simulink model "GS_model"  (R2018b)
settings: Solver=ode5  StartTime=0.0  StopTime=SimuStopTime  FixedStep=T_Simu  RelTol=1e-3
InitFcn:
  | Initial
undefined symbols (not defined in the file or in its folder): Aba10, Aba20, aeroCIP2006_S, aeroCIP2006_X, aeroCIP2006_Y, Agl0, Ass_kS, Ass_n1, Ass_n2, Ass_n3, Ass_n4, Ass_Noise, Ass_R, Ass_Resolution, Ass_TmOrder, AssA_Fix_Abs, AssB_Fix_Abs, AssC_Fix_Abs, AssD_Fix_Abs, AssE_Fix_Aps, AssF_Fix_Aps, C, c_max, c_min, Cd, CenterOfFigNX, CenterOfFigNY, CenterOfFigNZ, CenterOfFigP1, CenterOfFigP2, CenterOfFigPX, CenterOfFigPY, CenterOfFigPZ, Cmu, Crou, DEG2RAD, DiscIntNeverNeededParam, Eg_Dir, Eg_F, Eg_PrepareTime, Eg_r_L_L, Fw_Abf, Fw_Hmax, Fw_J, Fw_Spd0, Fw_Tmax, git_hash_BaseLine, git_hash_Project, Gnss_Noise_Pos, Gnss_Noise_Vel, Gnss_PropgationTime, GyroA_Fix_Abg, GyroA_Noise, GyroB_Fix_Abg, GyroB_Noise, GyroC_Fix_Abg, GyroC_Noise, GyroD_Fix_Abg, GyroD_Noise, h ... (+94)
libraries: simulink x308, sharedutil x46, aerolibutil x37, sharedtransform x31, vrlib x14, aerolibgravity2 x2
(part 7 of 20)

== system GS_model/Subsystem2/Subsystem/PhysicsModel/Environment/Air Torque Subsystem/Subsystem ==
  Sun Vector in J2000 : Inport
  Earth Vector in J2000 : Inport  Port=2
  Add : Sum
  Demux : Demux  Outputs=3
  Dot Product : DotProduct  InputSameDT=on  OutDataTypeStr=Inherit: Inherit via internal rule
  Dot Product1 : DotProduct  InputSameDT=on  OutDataTypeStr=Inherit: Inherit via internal rule
  Fcn : Fcn  Expr=sqrt(u(1)^2+u(2)^2)
  Gain : Gain  Gain=1e-9
  MATLAB Function : MATLAB Function  TreatAsAtomicUnit=on
  MATLAB Function1 : MATLAB Function  TreatAsAtomicUnit=on
  Math Function : Math  Operator=pow  SaturateOnIntegerOverflow=on
  Mux : Mux  Inputs=3
  Product : Product  Inputs=**/
  Product1 : Product  Inputs=**
  Product2 : Product  Inputs=**
  Product3 : Product  Inputs=**
  Saturation : Saturate  UpperLimit=2000000  LowerLimit=200000
  Sqrt : Sqrt  SaturateOnIntegerOverflow=on
  Terminator : Terminator
  Terminator1 : Terminator
  Trigonometric Function : Trigonometry  Operator=cos
  Trigonometric Function1 : Trigonometry
  Trigonometric Function2 : Trigonometry  Operator=cos
  Trigonometric Function3 : Trigonometry
  c_psi1 : Sum  Inputs=-+
  c_psi2 : Sum
  c_psi3 : Sum
  declination of sun : Trigonometry  Operator=atan2
  h : Constant  Value=h
  h1 : Constant  Value=c_min
  h2 : Constant  Value=c_max
  right ascension of sun : Trigonometry  Operator=atan2
  sun_delay : Constant  Value=ra_lag
  sun_delay2 : Constant  Value=0.5
  sun_delay3 : Constant  Value=n_prm
  rou : Outport
  wires:
  Demux/3 -> declination of sun/1
  Fcn/1 -> declination of sun/2
  Sun Vector in J2000/1 -> Fcn/1, Demux/1
  Demux/1 -> right ascension of sun/2
  Demux/2 -> right ascension of sun/1
  h2/1 -> MATLAB Function1/4(c_max)
  MATLAB Function/2(lat) -> Terminator1/1
  Product3/1 -> c_psi3/2
  Math Function/1 -> Product3/1
  c_psi3/1 -> Gain/1
  Gain/1 -> rou/1
  Product1/1 -> Mux/1
  c_psi2/1 -> Math Function/1
  Trigonometric Function1/1 -> Product2/1
  Sqrt/1 -> Product/3
  sun_delay2/1 -> c_psi2/1, Product/1
  Dot Product1/1 -> Sqrt/1
  Dot Product/1 -> Product/2
  MATLAB Function/3(h) -> Saturation/1
  Mux/1 -> Dot Product/1
  Saturation/1 -> MATLAB Function1/1(height)
  Trigonometric Function/1 -> Product1/1
  Trigonometric Function3/1 -> Mux/3
  Product2/1 -> Mux/2
  Trigonometric Function2/1 -> Product2/2, Product1/2
  MATLAB Function1/2(d_max) -> c_psi1/2
  MATLAB Function1/1(d_min) -> c_psi3/1, c_psi1/1
  c_psi1/1 -> Product3/2
  declination of sun/1 -> Trigonometric Function3/1, Trigonometric Function2/1
  Add/1 -> Trigonometric Function1/1, Trigonometric Function/1
  Product/1 -> c_psi2/2
  h/1 -> MATLAB Function1/2(h)
  h1/1 -> MATLAB Function1/3(c_min)
  sun_delay/1 -> Add/1
  right ascension of sun/1 -> Add/2
  sun_delay3/1 -> Math Function/2
  Earth Vector in J2000/1 -> Dot Product1/1, Dot Product/2, Dot Product1/2, MATLAB Function/1(r)
  MATLAB Function/1(lon) -> Terminator/1

== system GS_model/Subsystem2/Subsystem/PhysicsModel/Environment/Air Torque Subsystem/satalite board ==
  "[Vs]b" : Inport
  Fa' : Inport  Port=2
  Abp_PY : Inport  Port=3
  Abp_NY : Inport  Port=4
  Cent : Inport  Port=5
  UnlockSpread : Inport  Port=6
  +Y SolarPanel : Subsystem
  -Y SolarPanel : Subsystem
  Demux : Demux  Outputs=2
  Product{1..4} (4 alike) : Product  SaturateOnIntegerOverflow=on  OutDataTypeStr=Inherit: Same as first input
  Sum1 : Sum  Inputs=+++++
  Sum2 : Sum  Inputs=+++++
  "Torque from  board perpendicular to z axis " : Subsystem  TreatAsAtomicUnit=on
  Torque from board perpendicular to x axis : Subsystem  TreatAsAtomicUnit=on
  Torque from board perpendicular to y axis : Subsystem  TreatAsAtomicUnit=on
  F_a(b) : Outport
  T_a(b) : Outport  Port=2
  wires:
  "[Vs]b"/1 -> Torque from board perpendicular to x axis/1(vs(b)), Torque from board perpendicular to y axis/1(vs(b)), "Torque from  board perpendicular to z axis "/1("[Vs]b_nor"), +Y SolarPanel/1(vs(b)), -Y SolarPanel/1(vs(b))
  Fa'/1 -> Torque from board perpendicular to x axis/2(Fa'), Torque from board perpendicular to y axis/2(Fa'), "Torque from  board perpendicular to z axis "/2(Fa'), +Y SolarPanel/2(Fa'), -Y SolarPanel/2(Fa')
  Abp_PY/1 -> +Y SolarPanel/3("Abp ")
  Torque from board perpendicular to x axis/1(Tx) -> Sum1/1
  Sum1/1 -> T_a(b)/1
  Torque from board perpendicular to y axis/1(Ty) -> Sum1/2
  "Torque from  board perpendicular to z axis "/1(Tz) -> Sum1/3
  "Torque from  board perpendicular to z axis "/2(Fz) -> Sum2/3
  Torque from board perpendicular to y axis/2(Fy) -> Sum2/2
  Torque from board perpendicular to x axis/2(Fx) -> Sum2/1
  Sum2/1 -> F_a(b)/1
  Abp_NY/1 -> -Y SolarPanel/3("Abp ")
  Cent/1 -> Torque from board perpendicular to x axis/3(Cent), Torque from board perpendicular to y axis/3(Cent), +Y SolarPanel/4(Cent), -Y SolarPanel/4(Cent), "Torque from  board perpendicular to z axis "/3(Cent)
  Product2/1 -> Sum1/5
  Product4/1 -> Sum2/5
  +Y SolarPanel/2("F_panel ") -> Product3/1
  Product3/1 -> Sum2/4
  +Y SolarPanel/1("T_panel ") -> Product1/1
  Product1/1 -> Sum1/4
  -Y SolarPanel/1("T_panel ") -> Product2/2
  -Y SolarPanel/2("F_panel ") -> Product4/2
  UnlockSpread/1 -> Demux/1
  Demux/1 -> Product1/2, Product3/2
  Demux/2 -> Product4/1, Product2/1

== system GS_model/Subsystem2/Subsystem/PhysicsModel/Environment/MagneticCal/Subsystem1 ==
  LB_Geocentric : Inport
  Orbit : Inport  Port=2
  Aop1 : Subsystem
  Constant : Constant  Value=pi/2
  Divide : Product  Inputs=*/
  Fcn : Fcn  Expr=u(3)
  Fcn1 : Fcn  Expr=u(2)
  Fcn2 : Fcn  Expr=u(5)+u(6)
  Gain : Gain  Gain=-1
  If : If
  If Action Subsystem : Subsystem  TreatAsAtomicUnit=on
  If Action Subsystem1 : Subsystem  TreatAsAtomicUnit=on
  Merge : Merge
  Saturation : Saturate  UpperLimit=1  LowerLimit=-1
  Sum : Sum  Inputs=|-+
  Trigonometric Function : Trigonometry
  Trigonometric Function1 : Trigonometry  Operator=cos
  Trigonometric Function2 : Trigonometry  Operator=asin
  Trigonometric Function3 : Trigonometry  Operator=cos
  Aop : Outport
  wires:
  Trigonometric Function1/1 -> Gain/1
  Fcn/1 -> Trigonometric Function1/1  "i"
  Orbit/1 -> Fcn2/1, Fcn/1
  Constant/1 -> Sum/2
  Sum/1 -> Trigonometric Function/1
  Merge/1 -> Aop1/1(In1)
  Trigonometric Function/1 -> Divide/2
  If Action Subsystem1/1(Out1) -> Merge/2
  If/2 -> If Action Subsystem1/Action
  Fcn1/1 -> Sum/1
  If Action Subsystem/1(Out1) -> Merge/1
  Trigonometric Function3/1 -> If/1
  If/1 -> If Action Subsystem/Action
  Trigonometric Function2/1 -> If Action Subsystem1/1(In1), If Action Subsystem/1(In1)
  Fcn2/1 -> Trigonometric Function3/1  "u"
  Divide/1 -> Saturation/1
  Aop1/1(Out1) -> Aop/1
  Gain/1 -> Divide/1
  LB_Geocentric/1 -> Fcn1/1
  Saturation/1 -> Trigonometric Function2/1

== system GS_model/Subsystem2/Subsystem/PhysicsModel/Environment/Sun  press torque/Panel Angle ==
  Sun(b) : Inport
  Constant1 : Constant  Value=0
  Constant4 : Constant  Value=[0;0;-1]
  Demux : Demux  Outputs=3
  Divide1 : Product  Inputs=*/
  Dot Product : DotProduct  InputSameDT=on  OutDataTypeStr=Inherit: Inherit via internal rule
  Fcn2 : Fcn  Expr=sqrt(u(1)^2+u(2)^2+u(3)^2)
  Fcn3 : Fcn  Expr=u(1)
  If : If
  If Action Subsystem : Subsystem  TreatAsAtomicUnit=on
  If Action Subsystem1 : Subsystem  TreatAsAtomicUnit=on
  Merge : Merge
  Mux : Mux  Inputs=3
  Terminator : Terminator
  Trigonometric Function1 : Trigonometry  Operator=acos
  PanelAngle : Outport
  wires:
  Mux/1 -> Fcn2/1, Divide1/1
  Demux/3 -> Mux/3
  Constant1/1 -> Mux/2
  Demux/2 -> Terminator/1
  Demux/1 -> Mux/1
  Constant4/1 -> Dot Product/2
  Merge/1 -> PanelAngle/1
  Divide1/1 -> Fcn3/1, Dot Product/1
  Fcn3/1 -> If/1
  If/1 -> If Action Subsystem/Action
  If/2 -> If Action Subsystem1/Action
  If Action Subsystem/1(Out1) -> Merge/1
  If Action Subsystem1/1(Out1) -> Merge/2
  Fcn2/1 -> Divide1/2
  Trigonometric Function1/1 -> If Action Subsystem1/1(In1), If Action Subsystem/1(In1)
  Dot Product/1 -> Trigonometric Function1/1
  Sun(b)/1 -> Demux/1

== system GS_model/Subsystem2/Subsystem/PhysicsModel/Environment/Sun  press torque/Sun  press torque2 ==
  UnlockSpread : Inport
  Abp_PY : Inport  Port=2
  Abp_NY : Inport  Port=3
  Cent : Inport  Port=4
  IfSeeSun : Inport  Port=5
  TC_SunPressCoeff : Inport  Port=6
  Sun(b) : Inport  Port=7
  If Action Subsystem3 : Subsystem  TreatAsAtomicUnit=on
  If1 : If  IfExpression=u1 ==1
  Merge1 : Merge
  Merge3 : Merge
  Sun  press torque : Subsystem  TreatAsAtomicUnit=on
  F_sun : Outport
  T_sun : Outport  Port=2
  wires:
  If1/1 -> Sun  press torque/Action
  If1/2 -> If Action Subsystem3/Action
  Sun(b)/1 -> Sun  press torque/1(sun(b))
  Abp_PY/1 -> Sun  press torque/2(Abp_PY)
  If Action Subsystem3/2(T_sun) -> Merge3/2
  Sun  press torque/1(T_sun) -> Merge3/1
  Sun  press torque/2(F_sun) -> Merge1/1
  If Action Subsystem3/1(F_sun) -> Merge1/2
  Merge1/1 -> F_sun/1
  Merge3/1 -> T_sun/1
  IfSeeSun/1 -> If1/1
  Abp_NY/1 -> Sun  press torque/3(Abp_NY)
  Cent/1 -> Sun  press torque/4(Cent)
  UnlockSpread/1 -> Sun  press torque/5(UnlockSpread)
  TC_SunPressCoeff/1 -> Sun  press torque/6(TC_SunPressCoeff)

== system GS_model/Subsystem2/Subsystem/PhysicsModel/Environment/SunshineAreaCal/If Action Subsystem2 ==
  Action Port : ActionPort  ActionType=then
  Constant : Constant  Value=0
  Shadow : Outport  InitialOutput=0
  wires:
  Constant/1 -> Shadow/1

== system GS_model/Subsystem2/Subsystem/PhysicsModel/Environment/SunshineAreaCal/If Action Subsystem5 ==
  Action Port : ActionPort  ActionType=else
  Constant : Constant
  Sunshine : Outport  InitialOutput=1
  wires:
  Constant/1 -> Sunshine/1

== system GS_model/Subsystem2/Subsystem/PhysicsModel/Orbit/Compute osculating elements/  ==
  note: 0<=OMG<=2pi
  Hi : Inport
  Constant : Constant  Value=0
  Constant1 : Constant  Value=[1;0;0]
  Fcn1 : Fcn  Expr=u(1)
  Fcn2 : Fcn  Expr=u(2)
  If : If  IfExpression=u1 < 0
  If Action Subsystem : Subsystem  TreatAsAtomicUnit=on
  If Action Subsystem1 : Subsystem  TreatAsAtomicUnit=on
  MatrixMultiply : Product  Multiplication=Matrix(*)
  Merge : Merge
  Mux : Mux  Inputs=3
  Mux3 : Mux  Inputs=2
  Rotation Angles to Direction Cosine Matrix : sharedtransform/Rotation Angles to Direction Cosine Matrix  rotationOrder=ZYX  aMode=aMode
      settings: SourceProductBaseCode=AE,PW,MT,VE,VP
  Transpose : Math  Operator=transpose  SaturateOnIntegerOverflow=on
  tg(OMG)=Hxi/(-Hyi) : Fcn  Expr=atan2(u[1],-u[2])
  OMG : Outport
  N : Outport  Port=2
  wires:
  Fcn1/1 -> Mux3/1
  Fcn2/1 -> Mux3/2
  Mux3/1 -> tg(OMG)=Hxi/(-Hyi)/1
  tg(OMG)=Hxi/(-Hyi)/1 -> If/1, If Action Subsystem/1(In1), Mux/1, If Action Subsystem1/1(In1)
  If/1 -> If Action Subsystem/Action
  If/2 -> If Action Subsystem1/Action
  If Action Subsystem/1(Out1) -> Merge/1
  If Action Subsystem1/1(Out1) -> Merge/2
  Merge/1 -> OMG/1
  Hi/1 -> Fcn1/1, Fcn2/1
  Constant/1 -> Mux/2, Mux/3
  Mux/1 -> Rotation Angles to Direction Cosine Matrix/1
  Rotation Angles to Direction Cosine Matrix/1 -> Transpose/1
  Constant1/1 -> MatrixMultiply/2
  MatrixMultiply/1 -> N/1
  Transpose/1 -> MatrixMultiply/1

== system GS_model/Subsystem2/Subsystem/PhysicsModel/Orbit/Compute osculating elements/      ==
  N : Inport
  R_xyz : Inport  Port=2
  Divide : Product  Inputs=*/
  Dot Product4 : DotProduct  InputSameDT=on  OutDataTypeStr=Inherit: Inherit via internal rule
  Fcn3 : Fcn  Expr=sqrt(u[1]^2+u[2]^2+u[3]^2)
  Fcn4 : Fcn  Expr=u[3]
  If Action Subsystem2 : Subsystem  TreatAsAtomicUnit=on
  If Action Subsystem3 : Subsystem  TreatAsAtomicUnit=on
  If1 : If
  Merge1 : Merge
  Trigonometric Function : Trigonometry  Operator=acos
  u : Outport
  wires:
  N/1 -> Dot Product4/1
  R_xyz/1 -> Fcn3/1, Dot Product4/2, Fcn4/1
  Divide/1 -> Trigonometric Function/1
  Fcn4/1 -> If1/1
  If1/1 -> If Action Subsystem2/Action
  Trigonometric Function/1 -> If Action Subsystem2/1(In1), If Action Subsystem3/1(In1)
  If Action Subsystem2/1(Out1) -> Merge1/1
  If Action Subsystem3/1(Out1) -> Merge1/2
  Merge1/1 -> u/1
  If1/2 -> If Action Subsystem3/Action
  Dot Product4/1 -> Divide/1
  Fcn3/1 -> Divide/2

== system GS_model/Subsystem2/Subsystem/PhysicsModel/Orbit/Compute osculating elements/   1 ==
  note: e
  note: 0<=omg<=2pi
  H_xyz : Inport
  V_xyz : Inport  Port=2
  R_xyz : Inport  Port=3
  OMG : Inport  Port=4
  i : Inport  Port=5
  3x3 Cross Product1 : sharedutil/3x3 Cross Product  aMode=aMode
      settings: SourceProductBaseCode=AE,PW,MT,VE,VP
  Constant1 : Constant  Value=0
  Demux : Demux  Outputs=3
  Divide : Product  Inputs=*/
  Fcn3 : Fcn  Expr=sqrt(u[1]^2+u[2]^2+u[3]^2)
  Gain3 : Gain  Gain=1/miu  SaturateOnIntegerOverflow=on  OutDataTypeStr=Inherit: Same as input  ParamDataTypeStr=Inherit: Same as input
  If : If  IfExpression=u1 >= 0
  If Action Subsystem : Subsystem  TreatAsAtomicUnit=on
  If Action Subsystem1 : Subsystem  TreatAsAtomicUnit=on
  MatrixMultiply : Product  Multiplication=Matrix(*)
  Merge : Merge
  Mux1 : Mux  Inputs=3
  Rotation Angles to Direction Cosine Matrix : sharedtransform/Rotation Angles to Direction Cosine Matrix  rotationOrder=ZXY  aMode=aMode
      settings: SourceProductBaseCode=AE,PW,MT,VE,VP
  Sum : Sum  Inputs=|--  SaturateOnIntegerOverflow=on
  Terminator : Terminator
  Trigonometric Function : Trigonometry  Operator=atan2
  omg : Outport
  wires:
  H_xyz/1 -> 3x3 Cross Product1/1
  If Action Subsystem1/1(Out1) -> Merge/2
  If Action Subsystem/1(Out1) -> Merge/1
  Trigonometric Function/1 -> If/1, If Action Subsystem1/1(In1), If Action Subsystem/1(In1)
  Sum/1 -> MatrixMultiply/2
  Divide/1 -> Sum/2
  Fcn3/1 -> Divide/2
  3x3 Cross Product1/1 -> Gain3/1
  V_xyz/1 -> 3x3 Cross Product1/2
  Merge/1 -> omg/1
  If/1 -> If Action Subsystem/Action
  If/2 -> If Action Subsystem1/Action
  R_xyz/1 -> Divide/1, Fcn3/1
  Gain3/1 -> Sum/1
  Rotation Angles to Direction Cosine Matrix/1 -> MatrixMultiply/1
  Mux1/1 -> Rotation Angles to Direction Cosine Matrix/1
  OMG/1 -> Mux1/1
  i/1 -> Mux1/2
  Constant1/1 -> Mux1/3
  MatrixMultiply/1 -> Demux/1
  Demux/2 -> Trigonometric Function/1
  Demux/1 -> Trigonometric Function/2
  Demux/3 -> Terminator/1

== system GS_model/Subsystem2/Subsystem/Sensor/Ass/BodyAss(A&B&C&D)Model/Subsystem ==
  note: TC_AssGNDSet[6*1]
  note: TC_AssErr_Constant[2*1]
  note: TC_AssErr_WildValue[2*1]
  note: TC_AssErr_Jump[4*1]
  note: TC_AssErr_Wave[3*1]
  Sunshine : Inport
  AbAss : Inport  Port=2
  Sun_b : Inport  Port=3
  kS_Ass : Inport  Port=4
  TC_Ass : Inport  Port=5
  AssNum : Inport  Port=6
  AssErrModel : Subsystem
      mask Display: disp('AssErrModel')
  AssMathModel : Subsystem
      mask Display: disp('AssMathModel')
  Demux : Demux  Outputs=[6;2;2;4;3]
  TM_Data_AssA : Outport
  wires:
  Sunshine/1 -> AssMathModel/1(Sunshine)
  AbAss/1 -> AssMathModel/2(AbAss)
  Sun_b/1 -> AssMathModel/3(Sun_b)
  kS_Ass/1 -> AssMathModel/4(kS_Ass)
  AssMathModel/1(AssCur) -> AssErrModel/1(AssCur)
  Demux/1 -> AssErrModel/2(TC_AssGNDSet)
  Demux/2 -> AssErrModel/3(TC_AssErr_Constant)
  Demux/3 -> AssErrModel/4(TC_AssErr_WildValue)
  TC_Ass/1 -> Demux/1
  Demux/4 -> AssErrModel/5(TC_AssErr_Jump)
  Demux/5 -> AssErrModel/6(TC_AssErr_Wave)
  AssErrModel/1(TM_Ass_Cur) -> TM_Data_AssA/1
  AssNum/1 -> AssErrModel/7(AssNum)

== system GS_model/Subsystem2/Subsystem/Sensor/Ass/BodyAss(A&B&C&D)Model/Subsystem1 ==
  note: TC_AssErr_Wave[3*1]
  note: TC_AssErr_Jump[4*1]
  note: TC_AssErr_WildValue[2*1]
  note: TC_AssErr_Constant[2*1]
  note: TC_AssGNDSet[6*1]
  Sunshine : Inport
  AbAss : Inport  Port=2
  Sun_b : Inport  Port=3
  kS_Ass : Inport  Port=4
  TC_Ass : Inport  Port=5
  AssNum : Inport  Port=6
  AssErrModel : Subsystem
      mask Display: disp('AssErrModel')
  AssMathModel : Subsystem
      mask Display: disp('AssMathModel')
  Demux : Demux  Outputs=[6;2;2;4;3]
  TM_Data_AssA : Outport
  wires:
  AssNum/1 -> AssErrModel/7(AssNum)
  AssErrModel/1(TM_Ass_Cur) -> TM_Data_AssA/1
  Demux/5 -> AssErrModel/6(TC_AssErr_Wave)
  Demux/4 -> AssErrModel/5(TC_AssErr_Jump)
  TC_Ass/1 -> Demux/1
  Demux/3 -> AssErrModel/4(TC_AssErr_WildValue)
  Demux/2 -> AssErrModel/3(TC_AssErr_Constant)
  Demux/1 -> AssErrModel/2(TC_AssGNDSet)
  AssMathModel/1(AssCur) -> AssErrModel/1(AssCur)
  kS_Ass/1 -> AssMathModel/4(kS_Ass)
  Sun_b/1 -> AssMathModel/3(Sun_b)
  AbAss/1 -> AssMathModel/2(AbAss)
  Sunshine/1 -> AssMathModel/1(Sunshine)

== system GS_model/Subsystem2/Subsystem/Sensor/Ass/BodyAss(A&B&C&D)Model/Subsystem2 ==
  note: TC_AssGNDSet[6*1]
  note: TC_AssErr_Constant[2*1]
  note: TC_AssErr_WildValue[2*1]
  note: TC_AssErr_Jump[4*1]
  note: TC_AssErr_Wave[3*1]
  Sunshine : Inport
  AbAss : Inport  Port=2
  Sun_b : Inport  Port=3
  kS_Ass : Inport  Port=4
  TC_Ass : Inport  Port=5
  AssNum : Inport  Port=6
  AssErrModel : Subsystem
      mask Display: disp('AssErrModel')
  AssMathModel : Subsystem
      mask Display: disp('AssMathModel')
  Demux : Demux  Outputs=[6;2;2;4;3]
  TM_Data_AssA : Outport
  wires:
  Sunshine/1 -> AssMathModel/1(Sunshine)
  AbAss/1 -> AssMathModel/2(AbAss)
  Sun_b/1 -> AssMathModel/3(Sun_b)
  kS_Ass/1 -> AssMathModel/4(kS_Ass)
  AssMathModel/1(AssCur) -> AssErrModel/1(AssCur)
  Demux/1 -> AssErrModel/2(TC_AssGNDSet)
  Demux/2 -> AssErrModel/3(TC_AssErr_Constant)
  Demux/3 -> AssErrModel/4(TC_AssErr_WildValue)
  TC_Ass/1 -> Demux/1
  Demux/4 -> AssErrModel/5(TC_AssErr_Jump)
  Demux/5 -> AssErrModel/6(TC_AssErr_Wave)
  AssErrModel/1(TM_Ass_Cur) -> TM_Data_AssA/1
  AssNum/1 -> AssErrModel/7(AssNum)

== system GS_model/Subsystem2/Subsystem/Sensor/Ass/BodyAss(A&B&C&D)Model/Subsystem3 ==
  note: TC_AssErr_Wave[3*1]
  note: TC_AssErr_Jump[4*1]
  note: TC_AssErr_WildValue[2*1]
  note: TC_AssErr_Constant[2*1]
  note: TC_AssGNDSet[6*1]
  Sunshine : Inport
  AbAss : Inport  Port=2
  Sun_b : Inport  Port=3
  kS_Ass : Inport  Port=4
  TC_Ass : Inport  Port=5
  AssNum : Inport  Port=6
  AssErrModel : Subsystem
      mask Display: disp('AssErrModel')
  AssMathModel : Subsystem
      mask Display: disp('AssMathModel')
  Demux : Demux  Outputs=[6;2;2;4;3]
  TM_Data_AssA : Outport
  wires:
  AssNum/1 -> AssErrModel/7(AssNum)
  AssErrModel/1(TM_Ass_Cur) -> TM_Data_AssA/1
  Demux/5 -> AssErrModel/6(TC_AssErr_Wave)
  Demux/4 -> AssErrModel/5(TC_AssErr_Jump)
  TC_Ass/1 -> Demux/1
  Demux/3 -> AssErrModel/4(TC_AssErr_WildValue)
  Demux/2 -> AssErrModel/3(TC_AssErr_Constant)
  Demux/1 -> AssErrModel/2(TC_AssGNDSet)
  AssMathModel/1(AssCur) -> AssErrModel/1(AssCur)
  kS_Ass/1 -> AssMathModel/4(kS_Ass)
  Sun_b/1 -> AssMathModel/3(Sun_b)
  AbAss/1 -> AssMathModel/2(AbAss)
  Sunshine/1 -> AssMathModel/1(Sunshine)

== system GS_model/Subsystem2/Subsystem/Sensor/Ass/SolarPanelAss(E&F)Model/Subsystem ==
  note: TC_AssErr_Wave[3*1]
  note: TC_AssErr_Jump[4*1]
  note: TC_AssErr_WildValue[2*1]
  note: TC_AssErr_Constant[2*1]
  note: TC_AssGNDSet[6*1]
  Sunshine : Inport
  ApAss : Inport  Port=2
  Sun_b : Inport  Port=3
  kS_Ass : Inport  Port=4
  TC_Ass : Inport  Port=5
  Abp_PY : Inport  Port=6
  AssNum : Inport  Port=7
  AssErrModel : Subsystem
      mask Display: disp('AssErrModel')
  AssMathModel : Subsystem
      mask Display: disp('AssMathModel')
  Demux : Demux  Outputs=[6;2;2;4;3]
  TM_Data_AssE : Outport
  wires:
  AssErrModel/1(TM_Ass_Cur) -> TM_Data_AssE/1
  Demux/5 -> AssErrModel/6(TC_AssErr_Wave)
  Demux/4 -> AssErrModel/5(TC_AssErr_Jump)
  TC_Ass/1 -> Demux/1
  Demux/3 -> AssErrModel/4(TC_AssErr_WildValue)
  Demux/2 -> AssErrModel/3(TC_AssErr_Constant)
  Demux/1 -> AssErrModel/2(TC_AssGNDSet)
  AssMathModel/1(AssCur) -> AssErrModel/1(AssCur)
  kS_Ass/1 -> AssMathModel/4(kS_Ass)
  Sun_b/1 -> AssMathModel/3(Sun_b)
  ApAss/1 -> AssMathModel/2(ApAss)
  Sunshine/1 -> AssMathModel/1(Sunshine)
  Abp_PY/1 -> AssMathModel/5(Abp_PY)
  AssNum/1 -> AssErrModel/7(AssNum)

== system GS_model/Subsystem2/Subsystem/Sensor/Ass/SolarPanelAss(E&F)Model/Subsystem1 ==
  note: TC_AssGNDSet[6*1]
  note: TC_AssErr_Constant[2*1]
  note: TC_AssErr_WildValue[2*1]
  note: TC_AssErr_Jump[4*1]
  note: TC_AssErr_Wave[3*1]
  Sunshine : Inport
  ApAss : Inport  Port=2
  Sun_b : Inport  Port=3
  kS_Ass : Inport  Port=4
  TC_Ass : Inport  Port=5
  Abp_NY : Inport  Port=6
  AssNum : Inport  Port=7
  AssErrModel : Subsystem
      mask Display: disp('AssErrModel')
  AssMathModel : Subsystem
      mask Display: disp('AssMathModel')
  Demux : Demux  Outputs=[6;2;2;4;3]
  TM_Data_AssF : Outport
  wires:
  Abp_NY/1 -> AssMathModel/5(Abp_PY)
  Sunshine/1 -> AssMathModel/1(Sunshine)
  ApAss/1 -> AssMathModel/2(ApAss)
  Sun_b/1 -> AssMathModel/3(Sun_b)
  kS_Ass/1 -> AssMathModel/4(kS_Ass)
  AssMathModel/1(AssCur) -> AssErrModel/1(AssCur)
  Demux/1 -> AssErrModel/2(TC_AssGNDSet)
  Demux/2 -> AssErrModel/3(TC_AssErr_Constant)
  Demux/3 -> AssErrModel/4(TC_AssErr_WildValue)
  TC_Ass/1 -> Demux/1
  Demux/4 -> AssErrModel/5(TC_AssErr_Jump)
  Demux/5 -> AssErrModel/6(TC_AssErr_Wave)
  AssErrModel/1(TM_Ass_Cur) -> TM_Data_AssF/1
  AssNum/1 -> AssErrModel/7(AssNum)

== system GS_model/Subsystem2/Subsystem/Sensor/GNSS/GNSSErrModel/GNSSErrSet_Pos ==
  R_84 : Inport
  TC_GNSS_GNDSet_Pos : Inport  Port=2
  TC_GNSSErr_Pos_Constant : Inport  Port=3
  TC_GNSSErr_Pos_WildValue : Inport  Port=4
  Demux4 : Demux  Outputs=[1;3]
  GNSSErrSet_Constant : Subsystem
  GNSSErrSet_WildValue : Subsystem
  If : If  IfExpression=u1 == 1
  If Action Subsystem : Subsystem  TreatAsAtomicUnit=on
  If Action Subsystem1 : Subsystem  TreatAsAtomicUnit=on
  Merge : Merge
  TM_R_84 : Outport
  wires:
  R_84/1 -> GNSSErrSet_Constant/1(R_84_in)
  GNSSErrSet_Constant/1(R_84_out) -> GNSSErrSet_WildValue/1(R_84_in)
  TC_GNSSErr_Pos_Constant/1 -> GNSSErrSet_Constant/2(ErrSwitch)
  TC_GNSSErr_Pos_WildValue/1 -> GNSSErrSet_WildValue/2(ErrSwitch)
  Demux4/1 -> If/1
  Demux4/2 -> If Action Subsystem/1(In1)
  TC_GNSS_GNDSet_Pos/1 -> Demux4/1
  If/1 -> If Action Subsystem/Action
  GNSSErrSet_WildValue/1(R_84_out) -> If Action Subsystem1/1(In1)
  If/2 -> If Action Subsystem1/Action
  If Action Subsystem1/1(Out1) -> Merge/2
  If Action Subsystem/1(Out1) -> Merge/1
  Merge/1 -> TM_R_84/1

== system GS_model/Subsystem2/Subsystem/Sensor/GNSS/GNSSErrModel/GNSSErrSet_Pos1 ==
  TC_GNSS_GNDSet_Spd : Inport
  TC_GNSSErr_Spd_Constant : Inport  Port=2
  TC_GNSSErr_Spd_WildValue : Inport  Port=3
  V_84 : Inport  Port=4
  Demux4 : Demux  Outputs=[1;3]
  GNSSErrSet_Constant : Subsystem
  GNSSErrSet_WildValue : Subsystem
  If : If  IfExpression=u1 == 1
  If Action Subsystem : Subsystem  TreatAsAtomicUnit=on
  If Action Subsystem1 : Subsystem  TreatAsAtomicUnit=on
  Merge : Merge
  TM_V_84 : Outport
  wires:
  Merge/1 -> TM_V_84/1
  If Action Subsystem/1(Out1) -> Merge/1
  If Action Subsystem1/1(Out1) -> Merge/2
  If/2 -> If Action Subsystem1/Action
  GNSSErrSet_WildValue/1(V_84_out) -> If Action Subsystem1/1(In1)
  If/1 -> If Action Subsystem/Action
  TC_GNSS_GNDSet_Spd/1 -> Demux4/1
  Demux4/2 -> If Action Subsystem/1(In1)
  Demux4/1 -> If/1
  TC_GNSSErr_Spd_WildValue/1 -> GNSSErrSet_WildValue/2(ErrSwitch)
  TC_GNSSErr_Spd_Constant/1 -> GNSSErrSet_Constant/2(ErrSwitch)
  GNSSErrSet_Constant/1(V_84_out) -> GNSSErrSet_WildValue/1(V_84_in)
  V_84/1 -> GNSSErrSet_Constant/1(V_84_in)

== system GS_model/Subsystem2/Subsystem/Sensor/GNSS/Orbit/RV_i2RV_f1 ==
  R_i : Inport
  V_i : Inport  Port=2
  Afi : Inport  Port=3
  Constant : Constant  Value=[0;0;we]
  Cross Product : vrlib/Utilities/Cross Product
  MatrixMultiply : Product  Multiplication=Matrix(*)
  MatrixMultiply1 : Product  Multiplication=Matrix(*)
  Sum : Sum  Inputs=-+|
  R_f : Outport
  V_f : Outport  Port=2
  wires:
  MatrixMultiply/1 -> Cross Product/2, R_f/1
  Afi/1 -> MatrixMultiply/1, MatrixMultiply1/1
  R_i/1 -> MatrixMultiply/2
  V_i/1 -> MatrixMultiply1/2
  MatrixMultiply1/1 -> Sum/2
  Constant/1 -> Cross Product/1
  Cross Product/1 -> Sum/1
  Sum/1 -> V_f/1

== system GS_model/Subsystem2/Subsystem/Sensor/GNSS/Orbit/Subsystem1 ==
  UTC_1970 : Inport
  MATLAB Function : MATLAB Function  TreatAsAtomicUnit=on
  Afi : Outport
  wires:
  UTC_1970/1 -> MATLAB Function/1(Utc)
  MATLAB Function/1(A_GI) -> Afi/1

== system GS_model/Subsystem2/Subsystem/Sensor/GNSS/Orbit1/RV_i2RV_f1 ==
  R_i : Inport
  V_i : Inport  Port=2
  Afi : Inport  Port=3
  Constant : Constant  Value=[0;0;we]
  Cross Product : vrlib/Utilities/Cross Product
  MatrixMultiply : Product  Multiplication=Matrix(*)
  MatrixMultiply1 : Product  Multiplication=Matrix(*)
  Sum : Sum  Inputs=-+|
  R_f : Outport
  V_f : Outport  Port=2
  wires:
  Sum/1 -> V_f/1
  Cross Product/1 -> Sum/1
  Constant/1 -> Cross Product/1
  MatrixMultiply1/1 -> Sum/2
  V_i/1 -> MatrixMultiply1/2
  R_i/1 -> MatrixMultiply/2
  Afi/1 -> MatrixMultiply1/1, MatrixMultiply/1
  MatrixMultiply/1 -> R_f/1, Cross Product/2

== system GS_model/Subsystem2/Subsystem/Sensor/GNSS/Orbit1/Subsystem1 ==
  UTC_1970 : Inport
  MATLAB Function : MATLAB Function  TreatAsAtomicUnit=on
  Afi : Outport
  wires:
  MATLAB Function/1(A_GI) -> Afi/1
  UTC_1970/1 -> MATLAB Function/1(Utc)

== system GS_model/Subsystem2/Subsystem/Sensor/Gyro/GyroAModel/GyroErrSet ==
  note: TC_GyroGNDSet[5*1]
  note: TC_GyroErr_Constant[3*1]
  note: TC_GyroErr_WildValue[3*1]
  note: TC_GyroErr_Jump[5*1]
  note: TC_GyroErr_Wave[4*1]
  Wgi : Inport
  TC_Gyro : Inport  Port=2
  Gyro_Num : Inport  Port=3
  Constant : Constant  Value=0
  Constant2 : Constant  Value=0
  Demux : Demux  Outputs=[5;3;3;5;4]
  Demux1 : Demux  Outputs=[1;4]
  Demux10 : Demux  Outputs=[1;3]
  Demux2 : Demux  Outputs=[1;4]
  Demux3 : Demux  Outputs=[1;2]
  Demux6 : Demux  Outputs=[1;2]
  Demux8 : Demux  Outputs=[1;3]
  Gain : Gain  Gain=RAD2DEG
  GyroErrSet : Subsystem
  If Action Subsystem3 : Subsystem  TreatAsAtomicUnit=on
  If Action Subsystem4 : Subsystem  TreatAsAtomicUnit=on
  If1 : If  IfExpression=u1 == 1
  Logical Operator{,1..4} (5 alike) : Logic  Operator=OR  AllPortsSameDT=off  OutDataTypeStr=boolean
  Merge1 : Merge
  Relational Operator{1..10} (10 alike) : RelationalOperator  Operator===  OutDataTypeStr=boolean  RndMeth=Simplest
  Triggered Subsystem5 : Subsystem  TreatAsAtomicUnit=on
  Triggered Subsystem6 : Subsystem  TreatAsAtomicUnit=on
  Triggered Subsystem7 : Subsystem  TreatAsAtomicUnit=on
  Triggered Subsystem8 : Subsystem  TreatAsAtomicUnit=on
  Triggered Subsystem9 : Subsystem  TreatAsAtomicUnit=on
  TM_Gyro_Wgi : Outport
  wires:
  TC_Gyro/1 -> Demux/1
  Demux/1 -> Demux1/1
  Demux/2 -> Demux6/1
  Demux/4 -> Demux2/1
  Demux/5 -> Demux10/1
  Demux1/1 -> Relational Operator1/2, Relational Operator5/2
  Demux1/2 -> Triggered Subsystem6/1(In1)
  Gyro_Num/1 -> Relational Operator6/1, Relational Operator9/1, Relational Operator8/1, Relational Operator7/1, Relational Operator5/1
  Triggered Subsystem6/1(Out1) -> Demux8/1
  Demux8/1 -> If1/1
  If1/1 -> If Action Subsystem4/Action
  Demux8/2 -> If Action Subsystem4/1(In1)
  If Action Subsystem4/1(Out1) -> Merge1/1
  Merge1/1 -> Gain/1
  Demux10/2 -> Triggered Subsystem8/1(In1)
  Demux6/2 -> Triggered Subsystem9/1(In1)
  Demux2/2 -> Triggered Subsystem7/1(In1)
  GyroErrSet/1(Wgi_g) -> If Action Subsystem3/1(In1)
  If1/2 -> If Action Subsystem3/Action
  If Action Subsystem3/1(Out1) -> Merge1/2
  Wgi/1 -> GyroErrSet/1(Wgi)
  Triggered Subsystem9/1(Out1) -> GyroErrSet/2(TC_GyroErrSet_Constant)
  Triggered Subsystem5/1(Out1) -> GyroErrSet/3(TC_GyroErrSet_WildValue)
  Triggered Subsystem7/1(Out1) -> GyroErrSet/4(TC_GyroErrSet_Jump)
  Triggered Subsystem8/1(Out1) -> GyroErrSet/5(TC_StErrSet_Wave)
  Demux3/1 -> Relational Operator3/2, Relational Operator7/2
  Demux2/1 -> Relational Operator4/2, Relational Operator8/2
  Demux10/1 -> Relational Operator10/2, Relational Operator9/2
  Gain/1 -> TM_Gyro_Wgi/1
  Constant/1 -> Relational Operator1/1
  Relational Operator1/1 -> Logical Operator/1
  Relational Operator5/1 -> Logical Operator/2
  Logical Operator/1 -> Triggered Subsystem6/Enable
  Demux6/1 -> Relational Operator2/2, Relational Operator6/2
  Demux/3 -> Demux3/1
  Demux3/2 -> Triggered Subsystem5/1(In1)
  Relational Operator6/1 -> Logical Operator1/2
  Logical Operator1/1 -> Triggered Subsystem9/Enable
  Relational Operator2/1 -> Logical Operator1/1
  Constant2/1 -> Relational Operator10/1, Relational Operator4/1, Relational Operator3/1, Relational Operator2/1
  Logical Operator2/1 -> Triggered Subsystem5/Enable
  Relational Operator7/1 -> Logical Operator2/2
  Relational Operator3/1 -> Logical Operator2/1
  Relational Operator8/1 -> Logical Operator3/2
  Relational Operator4/1 -> Logical Operator3/1
  Logical Operator3/1 -> Triggered Subsystem7/Enable
  Relational Operator9/1 -> Logical Operator4/2
  Logical Operator4/1 -> Triggered Subsystem8/Enable
  Relational Operator10/1 -> Logical Operator4/1

== system GS_model/Subsystem2/Subsystem/Sensor/Gyro/GyroAModel/GyroMathModel ==
  note: Wgi(g) =Agb * ( Wbi(b) - Wbg(b) )
  Wbi_b : Inport
  Gyro_Fix_Abg : Inport  Port=2
  Gyro_Drift : Inport  Port=3
  Gyro_Noise : Inport  Port=4
  "Gyro_Num " : Inport  Port=5
  Constant : Constant  Value=0
  Demux2 : Demux  Outputs=[1;3]
  Logical Operator : Logic  Operator=OR  AllPortsSameDT=off  OutDataTypeStr=boolean
  Math Function : Math  Operator=transpose  SaturateOnIntegerOverflow=on
  Product : Product  Multiplication=Matrix(*)  RndMeth=Zero
  Relational Operator1 : RelationalOperator  Operator===  OutDataTypeStr=boolean  RndMeth=Simplest
  Relational Operator2 : RelationalOperator  Operator===  OutDataTypeStr=boolean  RndMeth=Simplest
  Sum : Sum  Inputs=+++
  Triggered Subsystem1 : Subsystem  TreatAsAtomicUnit=on
  Wgi_g : Outport
  wires:
  Gyro_Fix_Abg/1 -> Math Function/1
  Math Function/1 -> Product/1
  Gyro_Drift/1 -> Demux2/1  "TC_GyroDriftSet[4*1]"
  Product/1 -> Sum/1  "Wgi(g)"
  Sum/1 -> Wgi_g/1
  Wbi_b/1 -> Product/2
  Demux2/2 -> Triggered Subsystem1/1(In1)
  Triggered Subsystem1/1(Out1) -> Sum/2
  Gyro_Noise/1 -> Sum/3
  Demux2/1 -> Relational Operator2/2, Relational Operator1/2
  "Gyro_Num "/1 -> Relational Operator1/1
  Constant/1 -> Relational Operator2/1
  Relational Operator2/1 -> Logical Operator/1
  Relational Operator1/1 -> Logical Operator/2
  Logical Operator/1 -> Triggered Subsystem1/Enable

== system GS_model/Subsystem2/Subsystem/Sensor/Gyro/GyroBModel/GyroErrSet ==
  note: TC_GyroGNDSet[5*1]
  note: TC_GyroErr_Constant[3*1]
  note: TC_GyroErr_WildValue[3*1]
  note: TC_GyroErr_Jump[5*1]
  note: TC_GyroErr_Wave[4*1]
  Wgi : Inport
  TC_Gyro : Inport  Port=2
  Gyro_Num : Inport  Port=3
  Constant : Constant  Value=0
  Constant2 : Constant  Value=0
  Demux : Demux  Outputs=[5;3;3;5;4]
  Demux1 : Demux  Outputs=[1;4]
  Demux10 : Demux  Outputs=[1;3]
  Demux2 : Demux  Outputs=[1;4]
  Demux3 : Demux  Outputs=[1;2]
  Demux6 : Demux  Outputs=[1;2]
  Demux8 : Demux  Outputs=[1;3]
  Gain : Gain  Gain=RAD2DEG
  GyroErrSet : Subsystem
  If Action Subsystem3 : Subsystem  TreatAsAtomicUnit=on
  If Action Subsystem4 : Subsystem  TreatAsAtomicUnit=on
  If1 : If  IfExpression=u1 == 1
  Logical Operator{,1..4} (5 alike) : Logic  Operator=OR  AllPortsSameDT=off  OutDataTypeStr=boolean
  Merge1 : Merge
  Relational Operator{1..10} (10 alike) : RelationalOperator  Operator===  OutDataTypeStr=boolean  RndMeth=Simplest
  Triggered Subsystem5 : Subsystem  TreatAsAtomicUnit=on
  Triggered Subsystem6 : Subsystem  TreatAsAtomicUnit=on
  Triggered Subsystem7 : Subsystem  TreatAsAtomicUnit=on
  Triggered Subsystem8 : Subsystem  TreatAsAtomicUnit=on
  Triggered Subsystem9 : Subsystem  TreatAsAtomicUnit=on
  TM_Gyro_Wgi : Outport
  wires:
  TC_Gyro/1 -> Demux/1
  Demux/1 -> Demux1/1
  Demux/2 -> Demux6/1
  Demux/4 -> Demux2/1
  Demux/5 -> Demux10/1
  Demux1/1 -> Relational Operator1/2, Relational Operator5/2
  Demux1/2 -> Triggered Subsystem6/1(In1)
  Gyro_Num/1 -> Relational Operator6/1, Relational Operator9/1, Relational Operator8/1, Relational Operator7/1, Relational Operator5/1
  Triggered Subsystem6/1(Out1) -> Demux8/1
  Demux8/1 -> If1/1
  If1/1 -> If Action Subsystem4/Action
  Demux8/2 -> If Action Subsystem4/1(In1)
  If Action Subsystem4/1(Out1) -> Merge1/1
  Merge1/1 -> Gain/1
  Demux10/2 -> Triggered Subsystem8/1(In1)
  Demux6/2 -> Triggered Subsystem9/1(In1)
  Demux2/2 -> Triggered Subsystem7/1(In1)
  GyroErrSet/1(Wgi_g) -> If Action Subsystem3/1(In1)
  If1/2 -> If Action Subsystem3/Action
  If Action Subsystem3/1(Out1) -> Merge1/2
  Wgi/1 -> GyroErrSet/1(Wgi)
  Triggered Subsystem9/1(Out1) -> GyroErrSet/2(TC_GyroErrSet_Constant)
  Triggered Subsystem5/1(Out1) -> GyroErrSet/3(TC_GyroErrSet_WildValue)
  Triggered Subsystem7/1(Out1) -> GyroErrSet/4(TC_GyroErrSet_Jump)
  Triggered Subsystem8/1(Out1) -> GyroErrSet/5(TC_StErrSet_Wave)
  Demux3/1 -> Relational Operator3/2, Relational Operator7/2
  Demux2/1 -> Relational Operator4/2, Relational Operator8/2
  Demux10/1 -> Relational Operator10/2, Relational Operator9/2
  Gain/1 -> TM_Gyro_Wgi/1
  Constant/1 -> Relational Operator1/1
  Relational Operator1/1 -> Logical Operator/1
  Relational Operator5/1 -> Logical Operator/2
  Logical Operator/1 -> Triggered Subsystem6/Enable
  Demux6/1 -> Relational Operator2/2, Relational Operator6/2
  Demux/3 -> Demux3/1
  Demux3/2 -> Triggered Subsystem5/1(In1)
  Relational Operator6/1 -> Logical Operator1/2
  Logical Operator1/1 -> Triggered Subsystem9/Enable
  Relational Operator2/1 -> Logical Operator1/1
  Constant2/1 -> Relational Operator10/1, Relational Operator4/1, Relational Operator3/1, Relational Operator2/1
  Logical Operator2/1 -> Triggered Subsystem5/Enable
  Relational Operator7/1 -> Logical Operator2/2
  Relational Operator3/1 -> Logical Operator2/1
  Relational Operator8/1 -> Logical Operator3/2
  Relational Operator4/1 -> Logical Operator3/1
  Logical Operator3/1 -> Triggered Subsystem7/Enable
  Relational Operator9/1 -> Logical Operator4/2
  Logical Operator4/1 -> Triggered Subsystem8/Enable
  Relational Operator10/1 -> Logical Operator4/1

== system GS_model/Subsystem2/Subsystem/Sensor/Gyro/GyroBModel/GyroMathModel ==
  note: Wgi(g) =Agb * ( Wbi(b) - Wbg(b) )
  Wbi_b : Inport
  Gyro_Fix_Abg : Inport  Port=2
  Gyro_Drift : Inport  Port=3
  Gyro_Noise : Inport  Port=4
  "Gyro_Num " : Inport  Port=5
  Constant : Constant  Value=0
  Demux2 : Demux  Outputs=[1;3]
  Logical Operator : Logic  Operator=OR  AllPortsSameDT=off  OutDataTypeStr=boolean
  Math Function : Math  Operator=transpose  SaturateOnIntegerOverflow=on
  Product : Product  Multiplication=Matrix(*)  RndMeth=Zero
  Relational Operator1 : RelationalOperator  Operator===  OutDataTypeStr=boolean  RndMeth=Simplest
  Relational Operator2 : RelationalOperator  Operator===  OutDataTypeStr=boolean  RndMeth=Simplest
  Sum : Sum  Inputs=+++
  Triggered Subsystem1 : Subsystem  TreatAsAtomicUnit=on
  Wgi_g : Outport
  wires:
  Gyro_Fix_Abg/1 -> Math Function/1
  Math Function/1 -> Product/1
  Gyro_Drift/1 -> Demux2/1  "TC_GyroDriftSet[4*1]"
  Product/1 -> Sum/1  "Wgi(g)"
  Sum/1 -> Wgi_g/1
  Wbi_b/1 -> Product/2
  Demux2/2 -> Triggered Subsystem1/1(In1)
  Triggered Subsystem1/1(Out1) -> Sum/2
  Gyro_Noise/1 -> Sum/3
  Demux2/1 -> Relational Operator2/2, Relational Operator1/2
  "Gyro_Num "/1 -> Relational Operator1/1
  Constant/1 -> Relational Operator2/1
  Relational Operator2/1 -> Logical Operator/1
  Relational Operator1/1 -> Logical Operator/2
  Logical Operator/1 -> Triggered Subsystem1/Enable

== system GS_model/Subsystem2/Subsystem/Sensor/Gyro/GyroCModel/GyroErrSet ==
  note: TC_GyroGNDSet[5*1]
  note: TC_GyroErr_Constant[3*1]
  note: TC_GyroErr_WildValue[3*1]
  note: TC_GyroErr_Jump[5*1]
  note: TC_GyroErr_Wave[4*1]
  Wgi : Inport
  TC_Gyro : Inport  Port=2
  Gyro_Num : Inport  Port=3
  Constant : Constant  Value=0
  Constant2 : Constant  Value=0
  Demux : Demux  Outputs=[5;3;3;5;4]
  Demux1 : Demux  Outputs=[1;4]
  Demux10 : Demux  Outputs=[1;3]
  Demux2 : Demux  Outputs=[1;4]
  Demux3 : Demux  Outputs=[1;2]
  Demux6 : Demux  Outputs=[1;2]
  Demux8 : Demux  Outputs=[1;3]
  Gain : Gain  Gain=RAD2DEG
  GyroErrSet : Subsystem
  If Action Subsystem3 : Subsystem  TreatAsAtomicUnit=on
  If Action Subsystem4 : Subsystem  TreatAsAtomicUnit=on
  If1 : If  IfExpression=u1 == 1
  Logical Operator{,1..4} (5 alike) : Logic  Operator=OR  AllPortsSameDT=off  OutDataTypeStr=boolean
  Merge1 : Merge
  Relational Operator{1..10} (10 alike) : RelationalOperator  Operator===  OutDataTypeStr=boolean  RndMeth=Simplest
  Triggered Subsystem5 : Subsystem  TreatAsAtomicUnit=on
  Triggered Subsystem6 : Subsystem  TreatAsAtomicUnit=on
  Triggered Subsystem7 : Subsystem  TreatAsAtomicUnit=on
  Triggered Subsystem8 : Subsystem  TreatAsAtomicUnit=on
  Triggered Subsystem9 : Subsystem  TreatAsAtomicUnit=on
  TM_Gyro_Wgi : Outport
  wires:
  TC_Gyro/1 -> Demux/1
  Demux/1 -> Demux1/1
  Demux/2 -> Demux6/1
  Demux/4 -> Demux2/1
  Demux/5 -> Demux10/1
  Demux1/1 -> Relational Operator1/2, Relational Operator5/2
  Demux1/2 -> Triggered Subsystem6/1(In1)
  Gyro_Num/1 -> Relational Operator6/1, Relational Operator9/1, Relational Operator8/1, Relational Operator7/1, Relational Operator5/1
  Triggered Subsystem6/1(Out1) -> Demux8/1
  Demux8/1 -> If1/1
  If1/1 -> If Action Subsystem4/Action
  Demux8/2 -> If Action Subsystem4/1(In1)
  If Action Subsystem4/1(Out1) -> Merge1/1
  Merge1/1 -> Gain/1
  Demux10/2 -> Triggered Subsystem8/1(In1)
  Demux6/2 -> Triggered Subsystem9/1(In1)
  Demux2/2 -> Triggered Subsystem7/1(In1)
  GyroErrSet/1(Wgi_g) -> If Action Subsystem3/1(In1)
  If1/2 -> If Action Subsystem3/Action
  If Action Subsystem3/1(Out1) -> Merge1/2
  Wgi/1 -> GyroErrSet/1(Wgi)
  Triggered Subsystem9/1(Out1) -> GyroErrSet/2(TC_GyroErrSet_Constant)
  Triggered Subsystem5/1(Out1) -> GyroErrSet/3(TC_GyroErrSet_WildValue)
  Triggered Subsystem7/1(Out1) -> GyroErrSet/4(TC_GyroErrSet_Jump)
  Triggered Subsystem8/1(Out1) -> GyroErrSet/5(TC_StErrSet_Wave)
  Demux3/1 -> Relational Operator3/2, Relational Operator7/2
  Demux2/1 -> Relational Operator4/2, Relational Operator8/2
  Demux10/1 -> Relational Operator10/2, Relational Operator9/2
  Gain/1 -> TM_Gyro_Wgi/1
  Constant/1 -> Relational Operator1/1
  Relational Operator1/1 -> Logical Operator/1
  Relational Operator5/1 -> Logical Operator/2
  Logical Operator/1 -> Triggered Subsystem6/Enable
  Demux6/1 -> Relational Operator2/2, Relational Operator6/2
  Demux/3 -> Demux3/1
  Demux3/2 -> Triggered Subsystem5/1(In1)
  Relational Operator6/1 -> Logical Operator1/2
  Logical Operator1/1 -> Triggered Subsystem9/Enable
  Relational Operator2/1 -> Logical Operator1/1
  Constant2/1 -> Relational Operator10/1, Relational Operator4/1, Relational Operator3/1, Relational Operator2/1
  Logical Operator2/1 -> Triggered Subsystem5/Enable
  Relational Operator7/1 -> Logical Operator2/2
  Relational Operator3/1 -> Logical Operator2/1
  Relational Operator8/1 -> Logical Operator3/2
  Relational Operator4/1 -> Logical Operator3/1
  Logical Operator3/1 -> Triggered Subsystem7/Enable
  Relational Operator9/1 -> Logical Operator4/2
  Logical Operator4/1 -> Triggered Subsystem8/Enable
  Relational Operator10/1 -> Logical Operator4/1

== system GS_model/Subsystem2/Subsystem/Sensor/Gyro/GyroCModel/GyroMathModel ==
  note: Wgi(g) =Agb * ( Wbi(b) - Wbg(b) )
  Wbi_b : Inport
  Gyro_Fix_Abg : Inport  Port=2
  Gyro_Drift : Inport  Port=3
  Gyro_Noise : Inport  Port=4
  "Gyro_Num " : Inport  Port=5
  Constant : Constant  Value=0
  Demux2 : Demux  Outputs=[1;3]
  Logical Operator : Logic  Operator=OR  AllPortsSameDT=off  OutDataTypeStr=boolean
  Math Function : Math  Operator=transpose  SaturateOnIntegerOverflow=on
  Product : Product  Multiplication=Matrix(*)  RndMeth=Zero
  Relational Operator1 : RelationalOperator  Operator===  OutDataTypeStr=boolean  RndMeth=Simplest
  Relational Operator2 : RelationalOperator  Operator===  OutDataTypeStr=boolean  RndMeth=Simplest
  Sum : Sum  Inputs=+++
  Triggered Subsystem1 : Subsystem  TreatAsAtomicUnit=on
  Wgi_g : Outport
  wires:
  Gyro_Fix_Abg/1 -> Math Function/1
  Math Function/1 -> Product/1
  Gyro_Drift/1 -> Demux2/1  "TC_GyroDriftSet[4*1]"
  Product/1 -> Sum/1  "Wgi(g)"
  Sum/1 -> Wgi_g/1
  Wbi_b/1 -> Product/2
  Demux2/2 -> Triggered Subsystem1/1(In1)
  Triggered Subsystem1/1(Out1) -> Sum/2
  Gyro_Noise/1 -> Sum/3
  Demux2/1 -> Relational Operator2/2, Relational Operator1/2
  "Gyro_Num "/1 -> Relational Operator1/1
  Constant/1 -> Relational Operator2/1
  Relational Operator2/1 -> Logical Operator/1
  Relational Operator1/1 -> Logical Operator/2
  Logical Operator/1 -> Triggered Subsystem1/Enable

== system GS_model/Subsystem2/Subsystem/Sensor/Gyro/GyroDModel/GyroErrSet ==
  note: TC_GyroGNDSet[5*1]
  note: TC_GyroErr_Constant[3*1]
  note: TC_GyroErr_WildValue[3*1]
  note: TC_GyroErr_Jump[5*1]
  note: TC_GyroErr_Wave[4*1]
  Wgi : Inport
  TC_Gyro : Inport  Port=2
  Gyro_Num : Inport  Port=3
  Constant : Constant  Value=0
  Constant2 : Constant  Value=0
  Demux : Demux  Outputs=[5;3;3;5;4]
  Demux1 : Demux  Outputs=[1;4]
  Demux10 : Demux  Outputs=[1;3]
  Demux2 : Demux  Outputs=[1;4]
  Demux3 : Demux  Outputs=[1;2]
  Demux6 : Demux  Outputs=[1;2]
  Demux8 : Demux  Outputs=[1;3]
  Gain : Gain  Gain=RAD2DEG
  GyroErrSet : Subsystem
  If Action Subsystem3 : Subsystem  TreatAsAtomicUnit=on
  If Action Subsystem4 : Subsystem  TreatAsAtomicUnit=on
  If1 : If  IfExpression=u1 == 1
  Logical Operator{,1..4} (5 alike) : Logic  Operator=OR  AllPortsSameDT=off  OutDataTypeStr=boolean
  Merge1 : Merge
  Relational Operator{1..10} (10 alike) : RelationalOperator  Operator===  OutDataTypeStr=boolean  RndMeth=Simplest
  Triggered Subsystem5 : Subsystem  TreatAsAtomicUnit=on
  Triggered Subsystem6 : Subsystem  TreatAsAtomicUnit=on
  Triggered Subsystem7 : Subsystem  TreatAsAtomicUnit=on
  Triggered Subsystem8 : Subsystem  TreatAsAtomicUnit=on
  Triggered Subsystem9 : Subsystem  TreatAsAtomicUnit=on
  TM_Gyro_Wgi : Outport
  wires:
  TC_Gyro/1 -> Demux/1
  Demux/1 -> Demux1/1
  Demux/2 -> Demux6/1
  Demux/4 -> Demux2/1
  Demux/5 -> Demux10/1
  Demux1/1 -> Relational Operator1/2, Relational Operator5/2
  Demux1/2 -> Triggered Subsystem6/1(In1)
  Gyro_Num/1 -> Relational Operator6/1, Relational Operator9/1, Relational Operator8/1, Relational Operator7/1, Relational Operator5/1
  Triggered Subsystem6/1(Out1) -> Demux8/1
  Demux8/1 -> If1/1
  If1/1 -> If Action Subsystem4/Action
  Demux8/2 -> If Action Subsystem4/1(In1)
  If Action Subsystem4/1(Out1) -> Merge1/1
  Merge1/1 -> Gain/1
  Demux10/2 -> Triggered Subsystem8/1(In1)
  Demux6/2 -> Triggered Subsystem9/1(In1)
  Demux2/2 -> Triggered Subsystem7/1(In1)
  GyroErrSet/1(Wgi_g) -> If Action Subsystem3/1(In1)
  If1/2 -> If Action Subsystem3/Action
  If Action Subsystem3/1(Out1) -> Merge1/2
  Wgi/1 -> GyroErrSet/1(Wgi)
  Triggered Subsystem9/1(Out1) -> GyroErrSet/2(TC_GyroErrSet_Constant)
  Triggered Subsystem5/1(Out1) -> GyroErrSet/3(TC_GyroErrSet_WildValue)
  Triggered Subsystem7/1(Out1) -> GyroErrSet/4(TC_GyroErrSet_Jump)
  Triggered Subsystem8/1(Out1) -> GyroErrSet/5(TC_StErrSet_Wave)
  Demux3/1 -> Relational Operator3/2, Relational Operator7/2
  Demux2/1 -> Relational Operator4/2, Relational Operator8/2
  Demux10/1 -> Relational Operator10/2, Relational Operator9/2
  Gain/1 -> TM_Gyro_Wgi/1
  Constant/1 -> Relational Operator1/1
  Relational Operator1/1 -> Logical Operator/1
  Relational Operator5/1 -> Logical Operator/2
  Logical Operator/1 -> Triggered Subsystem6/Enable
  Demux6/1 -> Relational Operator2/2, Relational Operator6/2
  Demux/3 -> Demux3/1
  Demux3/2 -> Triggered Subsystem5/1(In1)
  Relational Operator6/1 -> Logical Operator1/2
  Logical Operator1/1 -> Triggered Subsystem9/Enable
  Relational Operator2/1 -> Logical Operator1/1
  Constant2/1 -> Relational Operator10/1, Relational Operator4/1, Relational Operator3/1, Relational Operator2/1
  Logical Operator2/1 -> Triggered Subsystem5/Enable
  Relational Operator7/1 -> Logical Operator2/2
  Relational Operator3/1 -> Logical Operator2/1
  Relational Operator8/1 -> Logical Operator3/2
  Relational Operator4/1 -> Logical Operator3/1
  Logical Operator3/1 -> Triggered Subsystem7/Enable
  Relational Operator9/1 -> Logical Operator4/2
  Logical Operator4/1 -> Triggered Subsystem8/Enable
  Relational Operator10/1 -> Logical Operator4/1

== system GS_model/Subsystem2/Subsystem/Sensor/Gyro/GyroDModel/GyroMathModel ==
  note: Wgi(g) =Agb * ( Wbi(b) - Wbg(b) )
  Wbi_b : Inport
  Gyro_Fix_Abg : Inport  Port=2
  Gyro_Drift : Inport  Port=3
  Gyro_Noise : Inport  Port=4
  "Gyro_Num " : Inport  Port=5
  Constant : Constant  Value=0
  Demux2 : Demux  Outputs=[1;3]
  Logical Operator : Logic  Operator=OR  AllPortsSameDT=off  OutDataTypeStr=boolean
  Math Function : Math  Operator=transpose  SaturateOnIntegerOverflow=on
  Product : Product  Multiplication=Matrix(*)  RndMeth=Zero
  Relational Operator1 : RelationalOperator  Operator===  OutDataTypeStr=boolean  RndMeth=Simplest
  Relational Operator2 : RelationalOperator  Operator===  OutDataTypeStr=boolean  RndMeth=Simplest
  Sum : Sum  Inputs=+++
  Triggered Subsystem1 : Subsystem  TreatAsAtomicUnit=on
  Wgi_g : Outport
  wires:
  Gyro_Fix_Abg/1 -> Math Function/1
  Math Function/1 -> Product/1
  Gyro_Drift/1 -> Demux2/1  "TC_GyroDriftSet[4*1]"
  Product/1 -> Sum/1  "Wgi(g)"
  Sum/1 -> Wgi_g/1
  Wbi_b/1 -> Product/2
  Demux2/2 -> Triggered Subsystem1/1(In1)
  Triggered Subsystem1/1(Out1) -> Sum/2
  Gyro_Noise/1 -> Sum/3
  Demux2/1 -> Relational Operator2/2, Relational Operator1/2
  "Gyro_Num "/1 -> Relational Operator1/1
  Constant/1 -> Relational Operator2/1
  Relational Operator2/1 -> Logical Operator/1
  Relational Operator1/1 -> Logical Operator/2
  Logical Operator/1 -> Triggered Subsystem1/Enable
